simulink model "untitled20210804"  (R2016b)
settings: Solver=ode4  StartTime=0.0  StopTime=inf  FixedStep=0.002  RelTol=1e-3  EnableMultiTasking=on
undefined symbols (not defined in the file or in its folder): bit, Standard
libraries: slrtlib x5, slrtsoftinglib x5
settings Model: xpc_rtwmakecfg_data=_xpccanac2pci_  SimulationMode=external  Creator=zczg  LastModifiedBy=zczg
settings SolverCC: EnableConcurrentExecution=on
settings DataIOCC: SaveFormat=StructureWithTime
settings OptimizationCC: BlockReduction=off  OptimizeBlockIOStorage=off  BufferReuse=off  GlobalBufferReuse=off  ExpressionFolding=off  LocalBlockOutputs=off
settings HardwareCC: ProdBitPerPointer=32  ProdBitPerSizeT=32  ProdBitPerPtrDiffT=32  ProdLargestAtomicFloat=None  ProdWordSize=32  ProdLongLongMode=on  ProdHWDeviceType=Generic->32-bit x86 compatible
settings RTWCC: SystemTargetFile=slrt.tlc  TemplateMakefile=slrt_default_tmf  Description=Simulink Real-Time  RTWCompilerOptimization=on

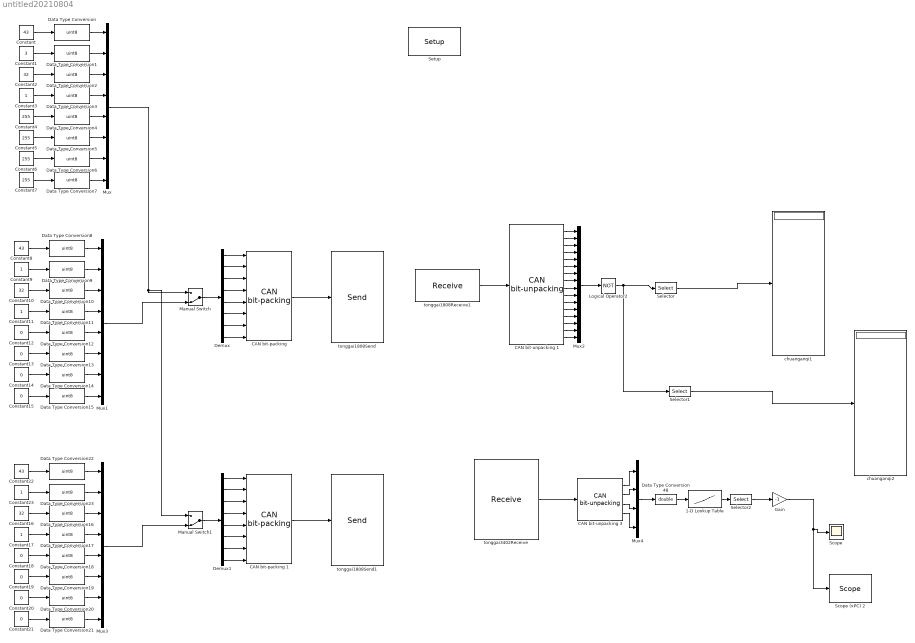
== system untitled20210804 ==
  1-D Lookup Table : Lookup_n-D  NumberOfTableDimensions=1  BreakpointsForDimension1=[3002 43350]  Table=[0 600]  InternalRulePriority=Speed  RndMeth=Simplest  InputSameDT=on
  "CAN bit-packing " : slrtlib/CAN/Utilities/CAN bit-packing   bitpatterns={ [0:7] [8:15] [16:23] [24:31] [32:39] [40:47] [48:55] [56:63]}
  CAN bit-packing 1 : slrtlib/CAN/Utilities/CAN bit-packing   bitpatterns={ [0:7] [8:15] [16:23] [24:31] [32:39] [40:47] [48:55] [56:63]}
  CAN bit-unpacking 1 : slrtlib/CAN/Utilities/CAN bit-unpacking   bitpatterns={0 1 2 3 4 5 6 7 8 9 10 11 12 13 14 15}  dtypes={ 'boolean','boolean','boolean','boolean','boolean','boolean','boolean','boolean','boolean','boolean','boolean','boolean','boolean','boolean','boolean','boolean'}
  CAN bit-unpacking 3 : slrtlib/CAN/Utilities/CAN bit-unpacking   bitpatterns={ [0:15],[16:31],[32:47],[48:63]}  dtypes={ 'uint16','uint16','uint16','uint16' }
  Constant : Constant  Value=43
  Constant1 : Constant  Value=3
  Constant10 : Constant  Value=32
  Constant{3,9,11,17,23} (5 alike) : Constant
  Constant{12..15,18..21} (8 alike) : Constant  Value=0
  Constant16 : Constant  Value=32
  Constant2 : Constant  Value=32
  Constant22 : Constant  Value=43
  Constant{4..7} (4 alike) : Constant  Value=255
  Constant8 : Constant  Value=43
  Data Type Conversion{,1..23} (24 alike) : DataTypeConversion  OutDataTypeStr=uint8
  Data Type Conversion48 : DataTypeConversion  OutDataTypeStr=double
  Demux : Demux  Outputs=8
  Demux1 : Demux  Outputs=8
  Gain : Gain  Gain=-1
  Logical Operator2 : Logic  Operator=NOT  AllPortsSameDT=off  OutDataTypeStr=boolean
  Manual Switch : ManualSwitch  CurrentSetting=0
  Manual Switch1 : ManualSwitch  CurrentSetting=0
  Mux : Mux  Inputs=8
  Mux1 : Mux  Inputs=8
  Mux2 : Mux  Inputs=16
  Mux3 : Mux  Inputs=8
  Mux4 : Mux
  Scope : Scope
  Scope (xPC) 2 : slrtlib/Displays and Logging/Scope   scopeno=3  scopetype=Target  autostart=on  viewmode=Numerical  formatstr='%15.6f'  grid=on  ylimits=[0,0]  nosamples=250  noprepostsamples=0  interleave=1  triggermode=FreeRun  triggersignal=1  trigsignalfromport=off  triggerlevel=0.0  triggerslope=Either  triggerscope=1  triggersample=0  filename=data.dat  mode=Lazy  writesize=512  autorestart=off  dynamicfilemode=off  maxwritefilesize=512*1024^2
  Selector : Selector  IndexOptions=Index vector (dialog)  Indices=[1:8]  OutputSizes=[(-2)]
  Selector1 : Selector  IndexOptions=Index vector (dialog)  Indices=[9:16]  OutputSizes=[(-2)]
  Selector2 : Selector  IndexOptions=Index vector (dialog)  Indices=[1]  OutputSizes=[(-2)]
  "Setup " : slrtsoftinglib/CAN-AC2-PCI SJA 1000/Setup   board=1  can1bus=Highspeed (ISO 11898)  can1Baudrate=500 kBaud  can1UserBR=[1,1,4,3]  can2bus=Highspeed (ISO 11898)  can2Baudrate=500 kBaud  can2UserBR=[1,1,4,3]  init=[]  term=[]  bus_off_out=off  bus_off_rec=Off  ioBaseAddress=-1
  chuanganqi1 : Display
  chuanganqi2 : Display
  tonggai1808Receive1 : slrtsoftinglib/CAN-AC2-PCI SJA 1000/Receive   board=1  canPort=CAN 1  range=Standard (11-bit)  ids=386  lengths=8  output=Data  inten=off  ts=-1  ididx=[1]
  tonggai1808Send : slrtsoftinglib/CAN-AC2-PCI SJA 1000/Send   board=1  canPort=CAN 1  range=Standard (11-bit)  ids=1538  sizes=[8]  output=off  ts=-1  ididx=[1]
  tonggai1808Send1 : slrtsoftinglib/CAN-AC2-PCI SJA 1000/Send   board=1  canPort=CAN 1  range=Standard (11-bit)  ids=1537  sizes=[8]  output=off  ts=-1  ididx=[0]
  tonggai3402Receive : slrtsoftinglib/CAN-AC2-PCI SJA 1000/Receive   board=1  canPort=CAN 1  range=Standard (11-bit)  ids=[385]  lengths=8  output=Data  inten=off  ts=-1  ididx=[0]
  wires:
  Data Type Conversion/1 -> Mux/1
  Data Type Conversion1/1 -> Mux/2
  Data Type Conversion2/1 -> Mux/3
  Data Type Conversion3/1 -> Mux/4
  Data Type Conversion4/1 -> Mux/5
  Data Type Conversion5/1 -> Mux/6
  Data Type Conversion6/1 -> Mux/7
  Data Type Conversion7/1 -> Mux/8
  Demux/1 -> "CAN bit-packing "/1
  Demux/2 -> "CAN bit-packing "/2
  Demux/3 -> "CAN bit-packing "/3
  Demux/4 -> "CAN bit-packing "/4
  Demux/5 -> "CAN bit-packing "/5
  Demux/6 -> "CAN bit-packing "/6
  Demux/7 -> "CAN bit-packing "/7
  Demux/8 -> "CAN bit-packing "/8
  "CAN bit-packing "/1 -> tonggai1808Send/1
  Constant/1 -> Data Type Conversion/1
  Constant1/1 -> Data Type Conversion1/1
  Constant2/1 -> Data Type Conversion2/1
  Constant3/1 -> Data Type Conversion3/1
  Constant4/1 -> Data Type Conversion4/1
  Constant5/1 -> Data Type Conversion5/1
  Constant6/1 -> Data Type Conversion6/1
  Constant7/1 -> Data Type Conversion7/1
  Data Type Conversion8/1 -> Mux1/1
  Data Type Conversion9/1 -> Mux1/2
  Data Type Conversion10/1 -> Mux1/3
  Data Type Conversion11/1 -> Mux1/4
  Data Type Conversion12/1 -> Mux1/5
  Data Type Conversion13/1 -> Mux1/6
  Data Type Conversion14/1 -> Mux1/7
  Data Type Conversion15/1 -> Mux1/8
  Constant8/1 -> Data Type Conversion8/1
  Constant9/1 -> Data Type Conversion9/1
  Constant10/1 -> Data Type Conversion10/1
  Constant11/1 -> Data Type Conversion11/1
  Constant12/1 -> Data Type Conversion12/1
  Constant13/1 -> Data Type Conversion13/1
  Constant14/1 -> Data Type Conversion14/1
  Constant15/1 -> Data Type Conversion15/1
  Manual Switch/1 -> Demux/1
  Mux/1 -> Manual Switch1/1, Manual Switch/1
  Mux1/1 -> Manual Switch/2
  Mux2/1 -> Logical Operator2/1
  tonggai1808Receive1/1 -> CAN bit-unpacking 1/1
  CAN bit-unpacking 1/1 -> Mux2/1
  CAN bit-unpacking 1/2 -> Mux2/2
  CAN bit-unpacking 1/3 -> Mux2/3
  CAN bit-unpacking 1/4 -> Mux2/4
  CAN bit-unpacking 1/5 -> Mux2/5
  CAN bit-unpacking 1/6 -> Mux2/6
  CAN bit-unpacking 1/7 -> Mux2/7
  CAN bit-unpacking 1/8 -> Mux2/8
  CAN bit-unpacking 1/9 -> Mux2/9
  CAN bit-unpacking 1/10 -> Mux2/10
  CAN bit-unpacking 1/11 -> Mux2/11
  CAN bit-unpacking 1/12 -> Mux2/12
  CAN bit-unpacking 1/13 -> Mux2/13
  CAN bit-unpacking 1/14 -> Mux2/14
  CAN bit-unpacking 1/15 -> Mux2/15
  CAN bit-unpacking 1/16 -> Mux2/16
  Logical Operator2/1 -> Selector1/1, Selector/1
  Selector/1 -> chuanganqi1/1
  Demux1/1 -> CAN bit-packing 1/1
  Demux1/2 -> CAN bit-packing 1/2
  Demux1/3 -> CAN bit-packing 1/3
  Demux1/4 -> CAN bit-packing 1/4
  Demux1/5 -> CAN bit-packing 1/5
  Demux1/6 -> CAN bit-packing 1/6
  Demux1/7 -> CAN bit-packing 1/7
  Demux1/8 -> CAN bit-packing 1/8
  CAN bit-packing 1/1 -> tonggai1808Send1/1
  Manual Switch1/1 -> Demux1/1
  Data Type Conversion22/1 -> Mux3/1
  Data Type Conversion23/1 -> Mux3/2
  Data Type Conversion16/1 -> Mux3/3
  Data Type Conversion17/1 -> Mux3/4
  Data Type Conversion18/1 -> Mux3/5
  Data Type Conversion19/1 -> Mux3/6
  Data Type Conversion20/1 -> Mux3/7
  Data Type Conversion21/1 -> Mux3/8
  Constant22/1 -> Data Type Conversion22/1
  Constant23/1 -> Data Type Conversion23/1
  Constant16/1 -> Data Type Conversion16/1
  Constant17/1 -> Data Type Conversion17/1
  Constant18/1 -> Data Type Conversion18/1
  Constant19/1 -> Data Type Conversion19/1
  Constant20/1 -> Data Type Conversion20/1
  Constant21/1 -> Data Type Conversion21/1
  Mux3/1 -> Manual Switch1/2
  CAN bit-unpacking 3/1 -> Mux4/1
  CAN bit-unpacking 3/2 -> Mux4/2
  CAN bit-unpacking 3/3 -> Mux4/3
  CAN bit-unpacking 3/4 -> Mux4/4
  Mux4/1 -> Data Type Conversion48/1
  tonggai3402Receive/1 -> CAN bit-unpacking 3/1
  Selector1/1 -> chuanganqi2/1
  Data Type Conversion48/1 -> 1-D Lookup Table/1
  1-D Lookup Table/1 -> Selector2/1
  Selector2/1 -> Gain/1
  Gain/1 -> Scope/1, Scope (xPC) 2/1
